simulink model "kwta2_block"  (R2024b)
settings: Solver=VariableStepAuto  StartTime=0.0  StopTime=2e-5  RelTol=1e-3
libraries: fl_lib x104, ee_lib x58, nesl_utility x13
(part 2 of 2)

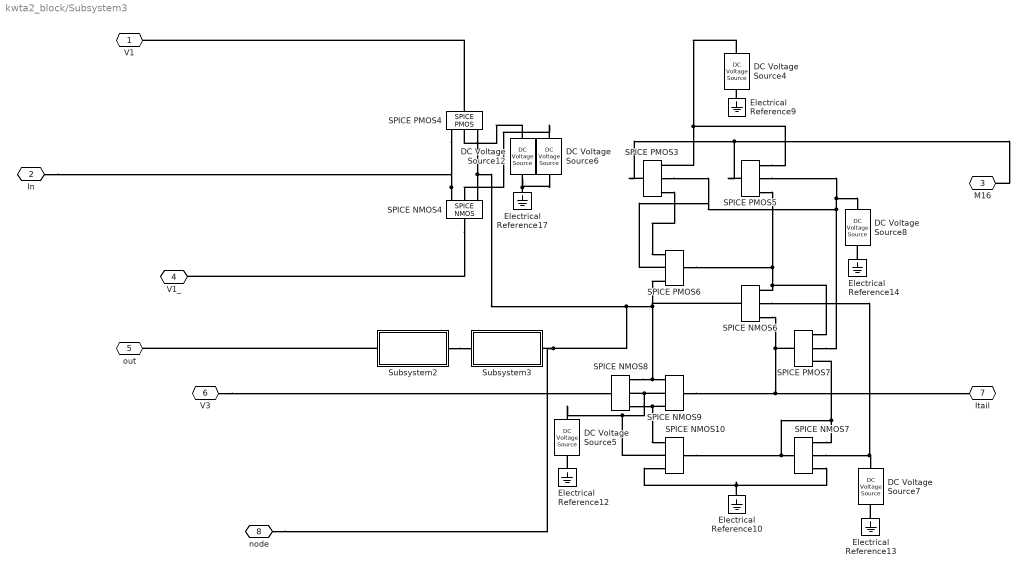
== system kwta2_block/Subsystem3 ==
  DC Voltage Source12 : fl_lib/Electrical/Electrical Sources/DC Voltage Source  v0=5 V
  DC Voltage Source4 : fl_lib/Electrical/Electrical Sources/DC Voltage Source  v0=5 V
  DC Voltage Source5 : fl_lib/Electrical/Electrical Sources/DC Voltage Source  v0=-5 V
  DC Voltage Source6 : fl_lib/Electrical/Electrical Sources/DC Voltage Source  v0=-5 V
  DC Voltage Source7 : fl_lib/Electrical/Electrical Sources/DC Voltage Source  v0=-5 V
  DC Voltage Source8 : fl_lib/Electrical/Electrical Sources/DC Voltage Source  v0=5 V
  Electrical Reference{9..10,12..14,17} (6 alike) : fl_lib/Electrical/Electrical Elements/Electrical Reference
  SPICE NMOS10 : ee_lib/Additional Components/SPICE Semiconductors/SPICE NMOS  LEVEL=3  AREA=1  SCALE=1  LENGTH=5 um  WIDTH=11 um  AD=0 m^2  AS=0 m^2  PD=0 m  PS=0 m  NRD=1  NRS=1  RD=0.01 Ohm  RS=1e-4 Ohm  RSH=NaN Ohm  VTO=0 V  KP=2e-5 A/V^2  GAMMA=0 V^0.50000  PHI=0.6 V  LAMBDA=0 1/V  IS=1e-14 A  N=1  JS=0 A/m^2  DELTA=0  VMAX=0 m/s  NFS=0 1/cm^2  ETA=0  THETA=0 1/V  KAPPA=0.2  Ci_param=ee.enum.intrinsicCapacitance.none  Cov_param=1  CGSO=0 F/m  CGDO=0 F/m  CGBO=0 F/m  C_param=1  CBD=0 F  CBS=0 F  PB=0.8 V  CJ=0 F/m^2  MJ=0.5  CJSW=0 F/m  MJSW=0.5  FC=0.5  IC_given=1  ICVDS=0 V  ICVGS=0 V  ICVBS=0 V  TOX=1e-7 m  LD=0 m  U0=600 cm^2/s/V  NSUB=NaN 1/cm^3  TPG=1  NSS=0 1/cm^2  XJ=0 m  T_param=1  TFIXED=300.15 K  TMEAS=300.15 K  TOFFSET=0 K  UEXP=0  UCRIT=1e+4 V/cm  NEFF=1  MTYPE=1
      settings: InternalSimscapePortConfiguration="{\"Bottom\":[],\"Left\":[{\"id\":\"gx\",\"label\":\"\",\"type\":\"foundation.electrical.electrical\"}],\"Right\":[{\"id\":\"dx\",\"label\":\"\",\"type\":\"foundation.electrical.electrical\"},{\"id\":\"bx\",\"label\":\"\",\"type\":\"foundation.electrical.electrical\"},{\"id\":\"sx\",\"label\":\"\",\"type\":\"foundation.electrical.electrical\"}],\"Top\":[]}"
  SPICE NMOS4 : ee_lib/Additional Components/SPICE Semiconductors/SPICE NMOS  LEVEL=3  AREA=1  SCALE=1  LENGTH=5 um  WIDTH=4 um  AD=0 m^2  AS=0 m^2  PD=0 m  PS=0 m  NRD=1  NRS=1  RD=0.01 Ohm  RS=1e-4 Ohm  RSH=NaN Ohm  VTO=0 V  KP=2e-5 A/V^2  GAMMA=0 V^0.50000  PHI=0.6 V  LAMBDA=0 1/V  IS=1e-14 A  N=1  JS=0 A/m^2  DELTA=0  VMAX=0 m/s  NFS=0 1/cm^2  ETA=0  THETA=0 1/V  KAPPA=0.2  Ci_param=ee.enum.intrinsicCapacitance.none  Cov_param=1  CGSO=0 F/m  CGDO=0 F/m  CGBO=0 F/m  C_param=1  CBD=0 F  CBS=0 F  PB=0.8 V  CJ=0 F/m^2  MJ=0.5  CJSW=0 F/m  MJSW=0.5  FC=0.5  IC_given=1  ICVDS=0 V  ICVGS=0 V  ICVBS=0 V  TOX=1e-7 m  LD=0 m  U0=600 cm^2/s/V  NSUB=NaN 1/cm^3  TPG=1  NSS=0 1/cm^2  XJ=0 m  T_param=1  TFIXED=300.15 K  TMEAS=300.15 K  TOFFSET=0 K  UEXP=0  UCRIT=1e+4 V/cm  NEFF=1  MTYPE=1
      settings: InternalSimscapePortConfiguration="{\"Bottom\":[],\"Left\":[{\"id\":\"gx\",\"label\":\"\",\"type\":\"foundation.electrical.electrical\"}],\"Right\":[{\"id\":\"dx\",\"label\":\"\",\"type\":\"foundation.electrical.electrical\"},{\"id\":\"bx\",\"label\":\"\",\"type\":\"foundation.electrical.electrical\"},{\"id\":\"sx\",\"label\":\"\",\"type\":\"foundation.electrical.electrical\"}],\"Top\":[]}"
  SPICE NMOS6 : ee_lib/Additional Components/SPICE Semiconductors/SPICE NMOS  LEVEL=3  AREA=1  SCALE=1  LENGTH=5 um  WIDTH=9 um  AD=0 m^2  AS=0 m^2  PD=0 m  PS=0 m  NRD=1  NRS=1  RD=0.01 Ohm  RS=1e-4 Ohm  RSH=NaN Ohm  VTO=0 V  KP=2e-5 A/V^2  GAMMA=0 V^0.50000  PHI=0.6 V  LAMBDA=0 1/V  IS=1e-14 A  N=1  JS=0 A/m^2  DELTA=0  VMAX=0 m/s  NFS=0 1/cm^2  ETA=0  THETA=0 1/V  KAPPA=0.2  Ci_param=ee.enum.intrinsicCapacitance.none  Cov_param=1  CGSO=0 F/m  CGDO=0 F/m  CGBO=0 F/m  C_param=1  CBD=0 F  CBS=0 F  PB=0.8 V  CJ=0 F/m^2  MJ=0.5  CJSW=0 F/m  MJSW=0.5  FC=0.5  IC_given=1  ICVDS=0 V  ICVGS=0 V  ICVBS=0 V  TOX=1e-7 m  LD=0 m  U0=600 cm^2/s/V  NSUB=NaN 1/cm^3  TPG=1  NSS=0 1/cm^2  XJ=0 m  T_param=1  TFIXED=300.15 K  TMEAS=300.15 K  TOFFSET=0 K  UEXP=0  UCRIT=1e+4 V/cm  NEFF=1  MTYPE=1
      settings: InternalSimscapePortConfiguration="{\"Bottom\":[],\"Left\":[{\"id\":\"gx\",\"label\":\"\",\"type\":\"foundation.electrical.electrical\"}],\"Right\":[{\"id\":\"dx\",\"label\":\"\",\"type\":\"foundation.electrical.electrical\"},{\"id\":\"bx\",\"label\":\"\",\"type\":\"foundation.electrical.electrical\"},{\"id\":\"sx\",\"label\":\"\",\"type\":\"foundation.electrical.electrical\"}],\"Top\":[]}"
  SPICE NMOS7 : ee_lib/Additional Components/SPICE Semiconductors/SPICE NMOS  LEVEL=3  AREA=1  SCALE=1  LENGTH=5 um  WIDTH=11 um  AD=0 m^2  AS=0 m^2  PD=0 m  PS=0 m  NRD=1  NRS=1  RD=0.01 Ohm  RS=1e-4 Ohm  RSH=NaN Ohm  VTO=0 V  KP=2e-5 A/V^2  GAMMA=0 V^0.50000  PHI=0.6 V  LAMBDA=0 1/V  IS=1e-14 A  N=1  JS=0 A/m^2  DELTA=0  VMAX=0 m/s  NFS=0 1/cm^2  ETA=0  THETA=0 1/V  KAPPA=0.2  Ci_param=ee.enum.intrinsicCapacitance.none  Cov_param=1  CGSO=0 F/m  CGDO=0 F/m  CGBO=0 F/m  C_param=1  CBD=0 F  CBS=0 F  PB=0.8 V  CJ=0 F/m^2  MJ=0.5  CJSW=0 F/m  MJSW=0.5  FC=0.5  IC_given=1  ICVDS=0 V  ICVGS=0 V  ICVBS=0 V  TOX=1e-7 m  LD=0 m  U0=600 cm^2/s/V  NSUB=NaN 1/cm^3  TPG=1  NSS=0 1/cm^2  XJ=0 m  T_param=1  TFIXED=300.15 K  TMEAS=300.15 K  TOFFSET=0 K  UEXP=0  UCRIT=1e+4 V/cm  NEFF=1  MTYPE=1
      settings: InternalSimscapePortConfiguration="{\"Bottom\":[],\"Left\":[{\"id\":\"gx\",\"label\":\"\",\"type\":\"foundation.electrical.electrical\"}],\"Right\":[{\"id\":\"dx\",\"label\":\"\",\"type\":\"foundation.electrical.electrical\"},{\"id\":\"bx\",\"label\":\"\",\"type\":\"foundation.electrical.electrical\"},{\"id\":\"sx\",\"label\":\"\",\"type\":\"foundation.electrical.electrical\"}],\"Top\":[]}"
  SPICE NMOS8 : ee_lib/Additional Components/SPICE Semiconductors/SPICE NMOS  LEVEL=3  AREA=1  SCALE=1  LENGTH=5 um  WIDTH=13 um  AD=0 m^2  AS=0 m^2  PD=0 m  PS=0 m  NRD=1  NRS=1  RD=0.01 Ohm  RS=1e-4 Ohm  RSH=NaN Ohm  VTO=0 V  KP=2e-5 A/V^2  GAMMA=0 V^0.50000  PHI=0.6 V  LAMBDA=0 1/V  IS=1e-14 A  N=1  JS=0 A/m^2  DELTA=0  VMAX=0 m/s  NFS=0 1/cm^2  ETA=0  THETA=0 1/V  KAPPA=0.2  Ci_param=ee.enum.intrinsicCapacitance.none  Cov_param=1  CGSO=0 F/m  CGDO=20 uF/m  CGBO=0 F/m  C_param=1  CBD=0 F  CBS=0 F  PB=0.8 V  CJ=0 F/m^2  MJ=0.5  CJSW=0 F/m  MJSW=0.5  FC=0.5  IC_given=1  ICVDS=0 V  ICVGS=0 V  ICVBS=0 V  TOX=1e-7 m  LD=0 m  U0=600 cm^2/s/V  NSUB=NaN 1/cm^3  TPG=1  NSS=0 1/cm^2  XJ=0 m  T_param=1  TFIXED=300.15 K  TMEAS=300.15 K  TOFFSET=0 K  UEXP=0  UCRIT=1e+4 V/cm  NEFF=1  MTYPE=1
      settings: InternalSimscapePortConfiguration="{\"Bottom\":[],\"Left\":[{\"id\":\"gx\",\"label\":\"\",\"type\":\"foundation.electrical.electrical\"}],\"Right\":[{\"id\":\"dx\",\"label\":\"\",\"type\":\"foundation.electrical.electrical\"},{\"id\":\"bx\",\"label\":\"\",\"type\":\"foundation.electrical.electrical\"},{\"id\":\"sx\",\"label\":\"\",\"type\":\"foundation.electrical.electrical\"}],\"Top\":[]}"
  SPICE NMOS9 : ee_lib/Additional Components/SPICE Semiconductors/SPICE NMOS  LEVEL=3  AREA=1  SCALE=1  LENGTH=5 um  WIDTH=13 um  AD=0 m^2  AS=0 m^2  PD=0 m  PS=0 m  NRD=1  NRS=1  RD=0.01 Ohm  RS=1e-4 Ohm  RSH=NaN Ohm  VTO=0 V  KP=2e-5 A/V^2  GAMMA=0 V^0.50000  PHI=0.6 V  LAMBDA=0 1/V  IS=1e-14 A  N=1  JS=0 A/m^2  DELTA=0  VMAX=0 m/s  NFS=0 1/cm^2  ETA=0  THETA=0 1/V  KAPPA=0.2  Ci_param=ee.enum.intrinsicCapacitance.none  Cov_param=2  CGSO=0 F/m  CGDO=1 uF/m  CGBO=0 F/m  C_param=2  CBD=0 F  CBS=0 F  PB=0.8 V  CJ=0 F/m^2  MJ=0.5  CJSW=0 F/m  MJSW=0.5  FC=0.5  IC_given=1  ICVDS=0 V  ICVGS=0 V  ICVBS=0 V  TOX=1e-7 m  LD=0 m  U0=600 cm^2/s/V  NSUB=NaN 1/cm^3  TPG=1  NSS=0 1/cm^2  XJ=0 m  T_param=1  TFIXED=300.15 K  TMEAS=300.15 K  TOFFSET=0 K  UEXP=0  UCRIT=1e+4 V/cm  NEFF=1  MTYPE=1
      settings: InternalSimscapePortConfiguration="{\"Bottom\":[],\"Left\":[{\"id\":\"gx\",\"label\":\"\",\"type\":\"foundation.electrical.electrical\"}],\"Right\":[{\"id\":\"dx\",\"label\":\"\",\"type\":\"foundation.electrical.electrical\"},{\"id\":\"bx\",\"label\":\"\",\"type\":\"foundation.electrical.electrical\"},{\"id\":\"sx\",\"label\":\"\",\"type\":\"foundation.electrical.electrical\"}],\"Top\":[]}"
  SPICE PMOS3 : ee_lib/Additional Components/SPICE Semiconductors/SPICE PMOS  LEVEL=3  AREA=1  SCALE=1  LENGTH=4 um  WIDTH=7 um  AD=0 m^2  AS=0 m^2  PD=0 m  PS=0 m  NRD=1  NRS=1  RD=0.01 Ohm  RS=1e-4 Ohm  RSH=NaN Ohm  VTO=0 V  KP=2e-5 A/V^2  GAMMA=0 V^0.50000  PHI=0.6 V  LAMBDA=0 1/V  IS=1e-14 A  N=1  JS=0 A/m^2  DELTA=0  VMAX=0 m/s  NFS=0 1/cm^2  ETA=0  THETA=0 1/V  KAPPA=0.2  Ci_param=ee.enum.intrinsicCapacitance.none  Cov_param=1  CGSO=0 F/m  CGDO=0 F/m  CGBO=0 F/m  C_param=1  CBD=0 F  CBS=0 F  PB=0.8 V  CJ=0 F/m^2  MJ=0.5  CJSW=0 F/m  MJSW=0.5  FC=0.5  IC_given=1  ICVDS=0 V  ICVGS=0 V  ICVBS=0 V  TOX=1e-7 m  LD=0 m  U0=600 cm^2/s/V  NSUB=NaN 1/cm^3  TPG=1  NSS=0 1/cm^2  XJ=0 m  T_param=1  TFIXED=300.15 K  TMEAS=300.15 K  TOFFSET=0 K  UEXP=0  UCRIT=1e+4 V/cm  NEFF=1  MTYPE=-1
      settings: InternalSimscapePortConfiguration="{\"Bottom\":[],\"Left\":[{\"id\":\"gx\",\"label\":\"\",\"type\":\"foundation.electrical.electrical\"}],\"Right\":[{\"id\":\"dx\",\"label\":\"\",\"type\":\"foundation.electrical.electrical\"},{\"id\":\"bx\",\"label\":\"\",\"type\":\"foundation.electrical.electrical\"},{\"id\":\"sx\",\"label\":\"\",\"type\":\"foundation.electrical.electrical\"}],\"Top\":[]}"
  SPICE PMOS4 : ee_lib/Additional Components/SPICE Semiconductors/SPICE PMOS  LEVEL=3  AREA=1  SCALE=1  LENGTH=5 um  WIDTH=4 um  AD=0 m^2  AS=0 m^2  PD=0 m  PS=0 m  NRD=1  NRS=1  RD=0.01 Ohm  RS=1e-4 Ohm  RSH=NaN Ohm  VTO=0 V  KP=2e-5 A/V^2  GAMMA=0 V^0.50000  PHI=0.6 V  LAMBDA=0 1/V  IS=1e-14 A  N=1  JS=0 A/m^2  DELTA=0  VMAX=0 m/s  NFS=0 1/cm^2  ETA=0  THETA=0 1/V  KAPPA=0.2  Ci_param=ee.enum.intrinsicCapacitance.none  Cov_param=1  CGSO=0 F/m  CGDO=0 F/m  CGBO=0 F/m  C_param=1  CBD=0 F  CBS=0 F  PB=0.8 V  CJ=0 F/m^2  MJ=0.5  CJSW=0 F/m  MJSW=0.5  FC=0.5  IC_given=1  ICVDS=0 V  ICVGS=0 V  ICVBS=0 V  TOX=1e-7 m  LD=0 m  U0=600 cm^2/s/V  NSUB=NaN 1/cm^3  TPG=1  NSS=0 1/cm^2  XJ=0 m  T_param=1  TFIXED=300.15 K  TMEAS=300.15 K  TOFFSET=0 K  UEXP=0  UCRIT=1e+4 V/cm  NEFF=1  MTYPE=-1
      settings: InternalSimscapePortConfiguration="{\"Bottom\":[],\"Left\":[{\"id\":\"gx\",\"label\":\"\",\"type\":\"foundation.electrical.electrical\"}],\"Right\":[{\"id\":\"dx\",\"label\":\"\",\"type\":\"foundation.electrical.electrical\"},{\"id\":\"bx\",\"label\":\"\",\"type\":\"foundation.electrical.electrical\"},{\"id\":\"sx\",\"label\":\"\",\"type\":\"foundation.electrical.electrical\"}],\"Top\":[]}"
  SPICE PMOS5 : ee_lib/Additional Components/SPICE Semiconductors/SPICE PMOS  LEVEL=3  AREA=1  SCALE=1  LENGTH=4 um  WIDTH=21 um  AD=0 m^2  AS=0 m^2  PD=0 m  PS=0 m  NRD=1  NRS=1  RD=0.01 Ohm  RS=1e-4 Ohm  RSH=NaN Ohm  VTO=0 V  KP=2e-5 A/V^2  GAMMA=0 V^0.50000  PHI=0.6 V  LAMBDA=0 1/V  IS=1e-14 A  N=1  JS=0 A/m^2  DELTA=0  VMAX=0 m/s  NFS=0 1/cm^2  ETA=0  THETA=0 1/V  KAPPA=0.2  Ci_param=ee.enum.intrinsicCapacitance.none  Cov_param=1  CGSO=0 F/m  CGDO=0 F/m  CGBO=0 F/m  C_param=1  CBD=0 F  CBS=0 F  PB=0.8 V  CJ=0 F/m^2  MJ=0.5  CJSW=0 F/m  MJSW=0.5  FC=0.5  IC_given=1  ICVDS=0 V  ICVGS=0 V  ICVBS=0 V  TOX=1e-7 m  LD=0 m  U0=600 cm^2/s/V  NSUB=NaN 1/cm^3  TPG=1  NSS=0 1/cm^2  XJ=0 m  T_param=1  TFIXED=300.15 K  TMEAS=300.15 K  TOFFSET=0 K  UEXP=0  UCRIT=1e+4 V/cm  NEFF=1  MTYPE=-1
      settings: InternalSimscapePortConfiguration="{\"Bottom\":[],\"Left\":[{\"id\":\"gx\",\"label\":\"\",\"type\":\"foundation.electrical.electrical\"}],\"Right\":[{\"id\":\"dx\",\"label\":\"\",\"type\":\"foundation.electrical.electrical\"},{\"id\":\"bx\",\"label\":\"\",\"type\":\"foundation.electrical.electrical\"},{\"id\":\"sx\",\"label\":\"\",\"type\":\"foundation.electrical.electrical\"}],\"Top\":[]}"
  SPICE PMOS6 : ee_lib/Additional Components/SPICE Semiconductors/SPICE PMOS  LEVEL=3  AREA=1  SCALE=1  LENGTH=4 um  WIDTH=7 um  AD=0 m^2  AS=0 m^2  PD=0 m  PS=0 m  NRD=1  NRS=1  RD=0.01 Ohm  RS=1e-4 Ohm  RSH=NaN Ohm  VTO=0 V  KP=2e-5 A/V^2  GAMMA=0 V^0.50000  PHI=0.6 V  LAMBDA=0 1/V  IS=1e-14 A  N=1  JS=0 A/m^2  DELTA=0  VMAX=0 m/s  NFS=0 1/cm^2  ETA=0  THETA=0 1/V  KAPPA=0.2  Ci_param=ee.enum.intrinsicCapacitance.none  Cov_param=1  CGSO=0 F/m  CGDO=0 F/m  CGBO=0 F/m  C_param=1  CBD=0 F  CBS=0 F  PB=0.8 V  CJ=0 F/m^2  MJ=0.5  CJSW=0 F/m  MJSW=0.5  FC=0.5  IC_given=1  ICVDS=0 V  ICVGS=0 V  ICVBS=0 V  TOX=1e-7 m  LD=0 m  U0=600 cm^2/s/V  NSUB=NaN 1/cm^3  TPG=1  NSS=0 1/cm^2  XJ=0 m  T_param=1  TFIXED=300.15 K  TMEAS=300.15 K  TOFFSET=0 K  UEXP=0  UCRIT=1e+4 V/cm  NEFF=1  MTYPE=-1
      settings: InternalSimscapePortConfiguration="{\"Bottom\":[],\"Left\":[{\"id\":\"gx\",\"label\":\"\",\"type\":\"foundation.electrical.electrical\"}],\"Right\":[{\"id\":\"dx\",\"label\":\"\",\"type\":\"foundation.electrical.electrical\"},{\"id\":\"bx\",\"label\":\"\",\"type\":\"foundation.electrical.electrical\"},{\"id\":\"sx\",\"label\":\"\",\"type\":\"foundation.electrical.electrical\"}],\"Top\":[]}"
  SPICE PMOS7 : ee_lib/Additional Components/SPICE Semiconductors/SPICE PMOS  LEVEL=3  AREA=1  SCALE=1  LENGTH=4 um  WIDTH=17 um  AD=0 m^2  AS=0 m^2  PD=0 m  PS=0 m  NRD=1  NRS=1  RD=0.01 Ohm  RS=1e-4 Ohm  RSH=NaN Ohm  VTO=0 V  KP=2e-5 A/V^2  GAMMA=0 V^0.50000  PHI=0.6 V  LAMBDA=0 1/V  IS=1e-14 A  N=1  JS=0 A/m^2  DELTA=0  VMAX=0 m/s  NFS=0 1/cm^2  ETA=0  THETA=0 1/V  KAPPA=0.2  Ci_param=ee.enum.intrinsicCapacitance.none  Cov_param=1  CGSO=0 F/m  CGDO=0 F/m  CGBO=0 F/m  C_param=1  CBD=0 F  CBS=0 F  PB=0.8 V  CJ=0 F/m^2  MJ=0.5  CJSW=0 F/m  MJSW=0.5  FC=0.5  IC_given=1  ICVDS=0 V  ICVGS=0 V  ICVBS=0 V  TOX=1e-7 m  LD=0 m  U0=600 cm^2/s/V  NSUB=NaN 1/cm^3  TPG=1  NSS=0 1/cm^2  XJ=0 m  T_param=1  TFIXED=300.15 K  TMEAS=300.15 K  TOFFSET=0 K  UEXP=0  UCRIT=1e+4 V/cm  NEFF=1  MTYPE=-1
      settings: InternalSimscapePortConfiguration="{\"Bottom\":[],\"Left\":[{\"id\":\"gx\",\"label\":\"\",\"type\":\"foundation.electrical.electrical\"}],\"Right\":[{\"id\":\"dx\",\"label\":\"\",\"type\":\"foundation.electrical.electrical\"},{\"id\":\"bx\",\"label\":\"\",\"type\":\"foundation.electrical.electrical\"},{\"id\":\"sx\",\"label\":\"\",\"type\":\"foundation.electrical.electrical\"}],\"Top\":[]}"
  Subsystem2 : Subsystem
  Subsystem3 : Subsystem
  V1 : PMIOPort  Side=Left
  In : PMIOPort  Port=2  Side=Left
  M16 : PMIOPort  Port=3  Side=Right
  V1_ : PMIOPort  Port=4  Side=Left
  out : PMIOPort  Port=5  Side=Left
  V3 : PMIOPort  Port=6  Side=Left
  Itail : PMIOPort  Port=7  Side=Right
  "node " : PMIOPort  Port=8  Side=Left
  connections:
  SPICE NMOS6/RConn3 -- Itail/RConn1 -- SPICE NMOS9/LConn1 -- SPICE PMOS7/LConn1
  SPICE PMOS5/RConn3 -- SPICE PMOS6/LConn1 -- SPICE PMOS7/RConn1 -- SPICE NMOS6/RConn1
  Electrical Reference10/LConn1 -- SPICE NMOS10/RConn3 -- SPICE NMOS7/RConn3
  Subsystem2/LConn1 -- out/RConn1
  DC Voltage Source4/LConn1 -- SPICE PMOS3/RConn1 -- SPICE PMOS5/RConn1
  DC Voltage Source6/LConn1 -- SPICE NMOS4/RConn2
  V3/RConn1 -- SPICE NMOS8/LConn1
  DC Voltage Source12/LConn1 -- SPICE PMOS4/RConn2
  DC Voltage Source5/LConn1 -- SPICE NMOS10/RConn2 -- SPICE NMOS9/RConn2 -- SPICE NMOS8/RConn2
  DC Voltage Source12/RConn1 -- DC Voltage Source6/RConn1 -- Electrical Reference17/LConn1
  SPICE NMOS4/RConn1 -- SPICE PMOS4/RConn3 -- In/RConn1
  SPICE PMOS5/LConn1 -- M16/RConn1 -- SPICE PMOS3/LConn1
  SPICE PMOS4/LConn1 -- V1/RConn1
  Electrical Reference9/LConn1 -- DC Voltage Source4/RConn1
  Electrical Reference14/LConn1 -- DC Voltage Source8/RConn1
  SPICE PMOS7/RConn2 -- SPICE PMOS3/RConn2 -- SPICE PMOS6/RConn2 -- SPICE PMOS5/RConn2 -- DC Voltage Source8/LConn1
  SPICE PMOS3/RConn3 -- SPICE PMOS6/RConn1
  SPICE NMOS10/LConn1 -- SPICE PMOS7/RConn3 -- SPICE NMOS7/RConn1 -- SPICE NMOS7/LConn1
  SPICE PMOS4/RConn1 -- SPICE NMOS4/RConn3 -- "node "/RConn1 -- Subsystem3/RConn1 -- SPICE PMOS6/RConn3 -- SPICE NMOS6/LConn1 -- SPICE NMOS8/RConn1 -- SPICE NMOS9/RConn1
  SPICE NMOS7/RConn2 -- SPICE NMOS6/RConn2 -- DC Voltage Source7/LConn1
  SPICE NMOS9/RConn3 -- SPICE NMOS8/RConn3 -- SPICE NMOS10/RConn1
  Subsystem2/RConn1 -- Subsystem3/LConn1
  SPICE NMOS4/LConn1 -- V1_/RConn1
  Electrical Reference13/LConn1 -- DC Voltage Source7/RConn1
  Electrical Reference12/LConn1 -- DC Voltage Source5/RConn1

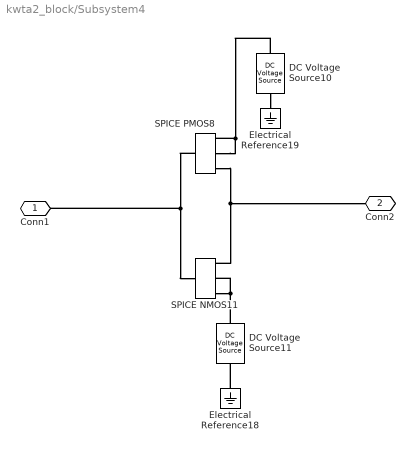
== system kwta2_block/Subsystem4 ==
  DC Voltage Source10 : fl_lib/Electrical/Electrical Sources/DC Voltage Source  v0=5 V
  DC Voltage Source11 : fl_lib/Electrical/Electrical Sources/DC Voltage Source  v0=0 V
  Electrical Reference18 : fl_lib/Electrical/Electrical Elements/Electrical Reference
  Electrical Reference19 : fl_lib/Electrical/Electrical Elements/Electrical Reference
  SPICE NMOS11 : ee_lib/Additional Components/SPICE Semiconductors/SPICE NMOS  LEVEL=1  AREA=1  SCALE=1  LENGTH=1e-4 mm  WIDTH=1e-4 mm  AD=0 m^2  AS=0 m^2  PD=0 m  PS=0 m  NRD=1  NRS=1  RD=0.01 Ohm  RS=1e-4 Ohm  RSH=NaN Ohm  VTO=0 V  KP=2e-5 A/V^2  GAMMA=0 V^0.50000  PHI=0.6 V  LAMBDA=0 1/V  IS=1e-14 A  N=1  JS=0 A/m^2  DELTA=0  VMAX=0 m/s  NFS=0 1/cm^2  ETA=0  THETA=0 1/V  KAPPA=0.2  Ci_param=ee.enum.intrinsicCapacitance.none  Cov_param=1  CGSO=0 F/m  CGDO=0 F/m  CGBO=0 F/m  C_param=1  CBD=0 F  CBS=0 F  PB=0.8 V  CJ=0 F/m^2  MJ=0.5  CJSW=0 F/m  MJSW=0.5  FC=0.5  IC_given=1  ICVDS=0 V  ICVGS=0 V  ICVBS=0 V  TOX=1e-7 m  LD=0 m  U0=600 cm^2/s/V  NSUB=NaN 1/cm^3  TPG=1  NSS=0 1/cm^2  XJ=0 m  T_param=1  TFIXED=300.15 K  TMEAS=300.15 K  TOFFSET=0 K  UEXP=0  UCRIT=1e+4 V/cm  NEFF=1  MTYPE=1
      settings: InternalSimscapePortConfiguration="{\"Bottom\":[],\"Left\":[{\"id\":\"gx\",\"label\":\"\",\"type\":\"foundation.electrical.electrical\"}],\"Right\":[{\"id\":\"dx\",\"label\":\"\",\"type\":\"foundation.electrical.electrical\"},{\"id\":\"bx\",\"label\":\"\",\"type\":\"foundation.electrical.electrical\"},{\"id\":\"sx\",\"label\":\"\",\"type\":\"foundation.electrical.electrical\"}],\"Top\":[]}"
  SPICE PMOS8 : ee_lib/Additional Components/SPICE Semiconductors/SPICE PMOS  LEVEL=1  AREA=1  SCALE=1  LENGTH=1e-4 mm  WIDTH=1e-4 mm  AD=0 m^2  AS=0 m^2  PD=0 m  PS=0 m  NRD=1  NRS=1  RD=0.01 Ohm  RS=1e-4 Ohm  RSH=NaN Ohm  VTO=0 V  KP=2e-5 A/V^2  GAMMA=0 V^0.50000  PHI=0.6 V  LAMBDA=0 1/V  IS=1e-14 A  N=1  JS=0 A/m^2  DELTA=0  VMAX=0 m/s  NFS=0 1/cm^2  ETA=0  THETA=0 1/V  KAPPA=0.2  Ci_param=ee.enum.intrinsicCapacitance.none  Cov_param=1  CGSO=0 F/m  CGDO=0 F/m  CGBO=0 F/m  C_param=1  CBD=0 F  CBS=0 F  PB=0.8 V  CJ=0 F/m^2  MJ=0.5  CJSW=0 F/m  MJSW=0.5  FC=0.5  IC_given=1  ICVDS=0 V  ICVGS=0 V  ICVBS=0 V  TOX=1e-7 m  LD=0 m  U0=600 cm^2/s/V  NSUB=NaN 1/cm^3  TPG=1  NSS=0 1/cm^2  XJ=0 m  T_param=1  TFIXED=300.15 K  TMEAS=300.15 K  TOFFSET=0 K  UEXP=0  UCRIT=1e+4 V/cm  NEFF=1  MTYPE=-1
      settings: InternalSimscapePortConfiguration="{\"Bottom\":[],\"Left\":[{\"id\":\"gx\",\"label\":\"\",\"type\":\"foundation.electrical.electrical\"}],\"Right\":[{\"id\":\"dx\",\"label\":\"\",\"type\":\"foundation.electrical.electrical\"},{\"id\":\"bx\",\"label\":\"\",\"type\":\"foundation.electrical.electrical\"},{\"id\":\"sx\",\"label\":\"\",\"type\":\"foundation.electrical.electrical\"}],\"Top\":[]}"
  Conn1 : PMIOPort  Side=Right
  Conn2 : PMIOPort  Port=2  Side=Left
  connections:
  DC Voltage Source10/RConn1 -- Electrical Reference19/LConn1
  SPICE NMOS11/RConn1 -- Conn2/RConn1 -- SPICE PMOS8/RConn3
  Electrical Reference18/LConn1 -- DC Voltage Source11/RConn1
  DC Voltage Source11/LConn1 -- SPICE NMOS11/RConn2 -- SPICE NMOS11/RConn3
  DC Voltage Source10/LConn1 -- SPICE PMOS8/RConn1 -- SPICE PMOS8/RConn2
  Conn1/RConn1 -- SPICE NMOS11/LConn1 -- SPICE PMOS8/LConn1

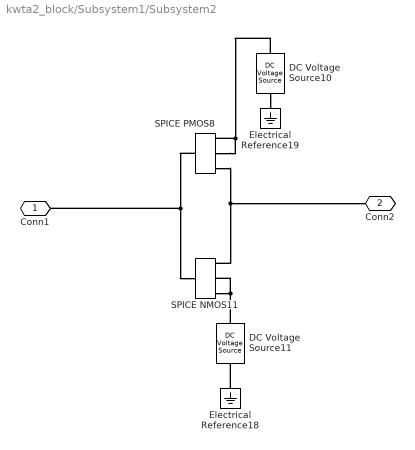
== system kwta2_block/Subsystem1/Subsystem2 ==
  DC Voltage Source10 : fl_lib/Electrical/Electrical Sources/DC Voltage Source  v0=5 V
  DC Voltage Source11 : fl_lib/Electrical/Electrical Sources/DC Voltage Source  v0=0 V
  Electrical Reference18 : fl_lib/Electrical/Electrical Elements/Electrical Reference
  Electrical Reference19 : fl_lib/Electrical/Electrical Elements/Electrical Reference
  SPICE NMOS11 : ee_lib/Additional Components/SPICE Semiconductors/SPICE NMOS  LEVEL=1  AREA=1  SCALE=1  LENGTH=1e-4 mm  WIDTH=1e-4 mm  AD=0 m^2  AS=0 m^2  PD=0 m  PS=0 m  NRD=1  NRS=1  RD=0.01 Ohm  RS=1e-4 Ohm  RSH=NaN Ohm  VTO=0 V  KP=2e-5 A/V^2  GAMMA=0 V^0.50000  PHI=0.6 V  LAMBDA=0 1/V  IS=1e-14 A  N=1  JS=0 A/m^2  DELTA=0  VMAX=0 m/s  NFS=0 1/cm^2  ETA=0  THETA=0 1/V  KAPPA=0.2  Ci_param=ee.enum.intrinsicCapacitance.none  Cov_param=1  CGSO=0 F/m  CGDO=0 F/m  CGBO=0 F/m  C_param=1  CBD=0 F  CBS=0 F  PB=0.8 V  CJ=0 F/m^2  MJ=0.5  CJSW=0 F/m  MJSW=0.5  FC=0.5  IC_given=1  ICVDS=0 V  ICVGS=0 V  ICVBS=0 V  TOX=1e-7 m  LD=0 m  U0=600 cm^2/s/V  NSUB=NaN 1/cm^3  TPG=1  NSS=0 1/cm^2  XJ=0 m  T_param=1  TFIXED=300.15 K  TMEAS=300.15 K  TOFFSET=0 K  UEXP=0  UCRIT=1e+4 V/cm  NEFF=1  MTYPE=1
      settings: InternalSimscapePortConfiguration="{\"Bottom\":[],\"Left\":[{\"id\":\"gx\",\"label\":\"\",\"type\":\"foundation.electrical.electrical\"}],\"Right\":[{\"id\":\"dx\",\"label\":\"\",\"type\":\"foundation.electrical.electrical\"},{\"id\":\"bx\",\"label\":\"\",\"type\":\"foundation.electrical.electrical\"},{\"id\":\"sx\",\"label\":\"\",\"type\":\"foundation.electrical.electrical\"}],\"Top\":[]}"
  SPICE PMOS8 : ee_lib/Additional Components/SPICE Semiconductors/SPICE PMOS  LEVEL=1  AREA=1  SCALE=1  LENGTH=1e-4 mm  WIDTH=1e-4 mm  AD=0 m^2  AS=0 m^2  PD=0 m  PS=0 m  NRD=1  NRS=1  RD=0.01 Ohm  RS=1e-4 Ohm  RSH=NaN Ohm  VTO=0 V  KP=2e-5 A/V^2  GAMMA=0 V^0.50000  PHI=0.6 V  LAMBDA=0 1/V  IS=1e-14 A  N=1  JS=0 A/m^2  DELTA=0  VMAX=0 m/s  NFS=0 1/cm^2  ETA=0  THETA=0 1/V  KAPPA=0.2  Ci_param=ee.enum.intrinsicCapacitance.none  Cov_param=1  CGSO=0 F/m  CGDO=0 F/m  CGBO=0 F/m  C_param=1  CBD=0 F  CBS=0 F  PB=0.8 V  CJ=0 F/m^2  MJ=0.5  CJSW=0 F/m  MJSW=0.5  FC=0.5  IC_given=1  ICVDS=0 V  ICVGS=0 V  ICVBS=0 V  TOX=1e-7 m  LD=0 m  U0=600 cm^2/s/V  NSUB=NaN 1/cm^3  TPG=1  NSS=0 1/cm^2  XJ=0 m  T_param=1  TFIXED=300.15 K  TMEAS=300.15 K  TOFFSET=0 K  UEXP=0  UCRIT=1e+4 V/cm  NEFF=1  MTYPE=-1
      settings: InternalSimscapePortConfiguration="{\"Bottom\":[],\"Left\":[{\"id\":\"gx\",\"label\":\"\",\"type\":\"foundation.electrical.electrical\"}],\"Right\":[{\"id\":\"dx\",\"label\":\"\",\"type\":\"foundation.electrical.electrical\"},{\"id\":\"bx\",\"label\":\"\",\"type\":\"foundation.electrical.electrical\"},{\"id\":\"sx\",\"label\":\"\",\"type\":\"foundation.electrical.electrical\"}],\"Top\":[]}"
  Conn1 : PMIOPort  Side=Right
  Conn2 : PMIOPort  Port=2  Side=Left
  connections:
  DC Voltage Source10/RConn1 -- Electrical Reference19/LConn1
  SPICE NMOS11/RConn1 -- Conn2/RConn1 -- SPICE PMOS8/RConn3
  Electrical Reference18/LConn1 -- DC Voltage Source11/RConn1
  DC Voltage Source11/LConn1 -- SPICE NMOS11/RConn2 -- SPICE NMOS11/RConn3
  DC Voltage Source10/LConn1 -- SPICE PMOS8/RConn1 -- SPICE PMOS8/RConn2
  Conn1/RConn1 -- SPICE NMOS11/LConn1 -- SPICE PMOS8/LConn1

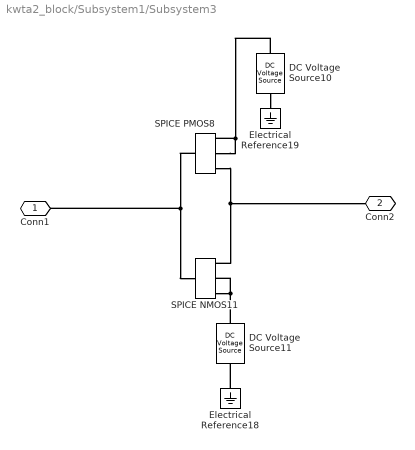
== system kwta2_block/Subsystem1/Subsystem3 ==
  DC Voltage Source10 : fl_lib/Electrical/Electrical Sources/DC Voltage Source  v0=5 V
  DC Voltage Source11 : fl_lib/Electrical/Electrical Sources/DC Voltage Source  v0=0 V
  Electrical Reference18 : fl_lib/Electrical/Electrical Elements/Electrical Reference
  Electrical Reference19 : fl_lib/Electrical/Electrical Elements/Electrical Reference
  SPICE NMOS11 : ee_lib/Additional Components/SPICE Semiconductors/SPICE NMOS  LEVEL=1  AREA=1  SCALE=1  LENGTH=1e-4 mm  WIDTH=1e-4 mm  AD=0 m^2  AS=0 m^2  PD=0 m  PS=0 m  NRD=1  NRS=1  RD=0.01 Ohm  RS=1e-4 Ohm  RSH=NaN Ohm  VTO=0 V  KP=2e-5 A/V^2  GAMMA=0 V^0.50000  PHI=0.6 V  LAMBDA=0 1/V  IS=1e-14 A  N=1  JS=0 A/m^2  DELTA=0  VMAX=0 m/s  NFS=0 1/cm^2  ETA=0  THETA=0 1/V  KAPPA=0.2  Ci_param=ee.enum.intrinsicCapacitance.none  Cov_param=1  CGSO=0 F/m  CGDO=0 F/m  CGBO=0 F/m  C_param=1  CBD=0 F  CBS=0 F  PB=0.8 V  CJ=0 F/m^2  MJ=0.5  CJSW=0 F/m  MJSW=0.5  FC=0.5  IC_given=1  ICVDS=0 V  ICVGS=0 V  ICVBS=0 V  TOX=1e-7 m  LD=0 m  U0=600 cm^2/s/V  NSUB=NaN 1/cm^3  TPG=1  NSS=0 1/cm^2  XJ=0 m  T_param=1  TFIXED=300.15 K  TMEAS=300.15 K  TOFFSET=0 K  UEXP=0  UCRIT=1e+4 V/cm  NEFF=1  MTYPE=1
      settings: InternalSimscapePortConfiguration="{\"Bottom\":[],\"Left\":[{\"id\":\"gx\",\"label\":\"\",\"type\":\"foundation.electrical.electrical\"}],\"Right\":[{\"id\":\"dx\",\"label\":\"\",\"type\":\"foundation.electrical.electrical\"},{\"id\":\"bx\",\"label\":\"\",\"type\":\"foundation.electrical.electrical\"},{\"id\":\"sx\",\"label\":\"\",\"type\":\"foundation.electrical.electrical\"}],\"Top\":[]}"
  SPICE PMOS8 : ee_lib/Additional Components/SPICE Semiconductors/SPICE PMOS  LEVEL=1  AREA=1  SCALE=1  LENGTH=1e-4 mm  WIDTH=1e-4 mm  AD=0 m^2  AS=0 m^2  PD=0 m  PS=0 m  NRD=1  NRS=1  RD=0.01 Ohm  RS=1e-4 Ohm  RSH=NaN Ohm  VTO=0 V  KP=2e-5 A/V^2  GAMMA=0 V^0.50000  PHI=0.6 V  LAMBDA=0 1/V  IS=1e-14 A  N=1  JS=0 A/m^2  DELTA=0  VMAX=0 m/s  NFS=0 1/cm^2  ETA=0  THETA=0 1/V  KAPPA=0.2  Ci_param=ee.enum.intrinsicCapacitance.none  Cov_param=1  CGSO=0 F/m  CGDO=0 F/m  CGBO=0 F/m  C_param=1  CBD=0 F  CBS=0 F  PB=0.8 V  CJ=0 F/m^2  MJ=0.5  CJSW=0 F/m  MJSW=0.5  FC=0.5  IC_given=1  ICVDS=0 V  ICVGS=0 V  ICVBS=0 V  TOX=1e-7 m  LD=0 m  U0=600 cm^2/s/V  NSUB=NaN 1/cm^3  TPG=1  NSS=0 1/cm^2  XJ=0 m  T_param=1  TFIXED=300.15 K  TMEAS=300.15 K  TOFFSET=0 K  UEXP=0  UCRIT=1e+4 V/cm  NEFF=1  MTYPE=-1
      settings: InternalSimscapePortConfiguration="{\"Bottom\":[],\"Left\":[{\"id\":\"gx\",\"label\":\"\",\"type\":\"foundation.electrical.electrical\"}],\"Right\":[{\"id\":\"dx\",\"label\":\"\",\"type\":\"foundation.electrical.electrical\"},{\"id\":\"bx\",\"label\":\"\",\"type\":\"foundation.electrical.electrical\"},{\"id\":\"sx\",\"label\":\"\",\"type\":\"foundation.electrical.electrical\"}],\"Top\":[]}"
  Conn1 : PMIOPort  Side=Right
  Conn2 : PMIOPort  Port=2  Side=Left
  connections:
  SPICE PMOS8/LConn1 -- SPICE NMOS11/LConn1 -- Conn1/RConn1
  SPICE PMOS8/RConn2 -- SPICE PMOS8/RConn1 -- DC Voltage Source10/LConn1
  SPICE NMOS11/RConn3 -- SPICE NMOS11/RConn2 -- DC Voltage Source11/LConn1
  Electrical Reference18/LConn1 -- DC Voltage Source11/RConn1
  SPICE PMOS8/RConn3 -- Conn2/RConn1 -- SPICE NMOS11/RConn1
  DC Voltage Source10/RConn1 -- Electrical Reference19/LConn1

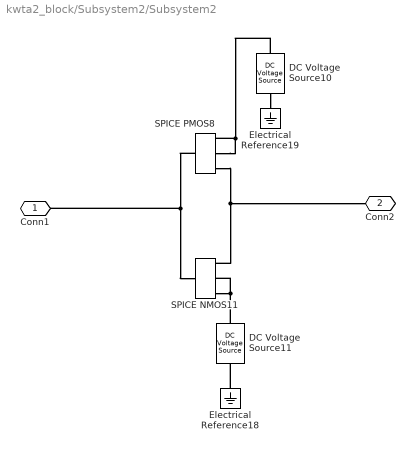
== system kwta2_block/Subsystem2/Subsystem2 ==
  DC Voltage Source10 : fl_lib/Electrical/Electrical Sources/DC Voltage Source  v0=5 V
  DC Voltage Source11 : fl_lib/Electrical/Electrical Sources/DC Voltage Source  v0=0 V
  Electrical Reference18 : fl_lib/Electrical/Electrical Elements/Electrical Reference
  Electrical Reference19 : fl_lib/Electrical/Electrical Elements/Electrical Reference
  SPICE NMOS11 : ee_lib/Additional Components/SPICE Semiconductors/SPICE NMOS  LEVEL=1  AREA=1  SCALE=1  LENGTH=1e-4 mm  WIDTH=1e-4 mm  AD=0 m^2  AS=0 m^2  PD=0 m  PS=0 m  NRD=1  NRS=1  RD=0.01 Ohm  RS=1e-4 Ohm  RSH=NaN Ohm  VTO=0 V  KP=2e-5 A/V^2  GAMMA=0 V^0.50000  PHI=0.6 V  LAMBDA=0 1/V  IS=1e-14 A  N=1  JS=0 A/m^2  DELTA=0  VMAX=0 m/s  NFS=0 1/cm^2  ETA=0  THETA=0 1/V  KAPPA=0.2  Ci_param=ee.enum.intrinsicCapacitance.none  Cov_param=1  CGSO=0 F/m  CGDO=0 F/m  CGBO=0 F/m  C_param=1  CBD=0 F  CBS=0 F  PB=0.8 V  CJ=0 F/m^2  MJ=0.5  CJSW=0 F/m  MJSW=0.5  FC=0.5  IC_given=1  ICVDS=0 V  ICVGS=0 V  ICVBS=0 V  TOX=1e-7 m  LD=0 m  U0=600 cm^2/s/V  NSUB=NaN 1/cm^3  TPG=1  NSS=0 1/cm^2  XJ=0 m  T_param=1  TFIXED=300.15 K  TMEAS=300.15 K  TOFFSET=0 K  UEXP=0  UCRIT=1e+4 V/cm  NEFF=1  MTYPE=1
      settings: InternalSimscapePortConfiguration="{\"Bottom\":[],\"Left\":[{\"id\":\"gx\",\"label\":\"\",\"type\":\"foundation.electrical.electrical\"}],\"Right\":[{\"id\":\"dx\",\"label\":\"\",\"type\":\"foundation.electrical.electrical\"},{\"id\":\"bx\",\"label\":\"\",\"type\":\"foundation.electrical.electrical\"},{\"id\":\"sx\",\"label\":\"\",\"type\":\"foundation.electrical.electrical\"}],\"Top\":[]}"
  SPICE PMOS8 : ee_lib/Additional Components/SPICE Semiconductors/SPICE PMOS  LEVEL=1  AREA=1  SCALE=1  LENGTH=1e-4 mm  WIDTH=1e-4 mm  AD=0 m^2  AS=0 m^2  PD=0 m  PS=0 m  NRD=1  NRS=1  RD=0.01 Ohm  RS=1e-4 Ohm  RSH=NaN Ohm  VTO=0 V  KP=2e-5 A/V^2  GAMMA=0 V^0.50000  PHI=0.6 V  LAMBDA=0 1/V  IS=1e-14 A  N=1  JS=0 A/m^2  DELTA=0  VMAX=0 m/s  NFS=0 1/cm^2  ETA=0  THETA=0 1/V  KAPPA=0.2  Ci_param=ee.enum.intrinsicCapacitance.none  Cov_param=1  CGSO=0 F/m  CGDO=0 F/m  CGBO=0 F/m  C_param=1  CBD=0 F  CBS=0 F  PB=0.8 V  CJ=0 F/m^2  MJ=0.5  CJSW=0 F/m  MJSW=0.5  FC=0.5  IC_given=1  ICVDS=0 V  ICVGS=0 V  ICVBS=0 V  TOX=1e-7 m  LD=0 m  U0=600 cm^2/s/V  NSUB=NaN 1/cm^3  TPG=1  NSS=0 1/cm^2  XJ=0 m  T_param=1  TFIXED=300.15 K  TMEAS=300.15 K  TOFFSET=0 K  UEXP=0  UCRIT=1e+4 V/cm  NEFF=1  MTYPE=-1
      settings: InternalSimscapePortConfiguration="{\"Bottom\":[],\"Left\":[{\"id\":\"gx\",\"label\":\"\",\"type\":\"foundation.electrical.electrical\"}],\"Right\":[{\"id\":\"dx\",\"label\":\"\",\"type\":\"foundation.electrical.electrical\"},{\"id\":\"bx\",\"label\":\"\",\"type\":\"foundation.electrical.electrical\"},{\"id\":\"sx\",\"label\":\"\",\"type\":\"foundation.electrical.electrical\"}],\"Top\":[]}"
  Conn1 : PMIOPort  Side=Right
  Conn2 : PMIOPort  Port=2  Side=Left
  connections:
  SPICE PMOS8/LConn1 -- SPICE NMOS11/LConn1 -- Conn1/RConn1
  SPICE PMOS8/RConn2 -- SPICE PMOS8/RConn1 -- DC Voltage Source10/LConn1
  SPICE NMOS11/RConn3 -- SPICE NMOS11/RConn2 -- DC Voltage Source11/LConn1
  Electrical Reference18/LConn1 -- DC Voltage Source11/RConn1
  SPICE PMOS8/RConn3 -- Conn2/RConn1 -- SPICE NMOS11/RConn1
  DC Voltage Source10/RConn1 -- Electrical Reference19/LConn1

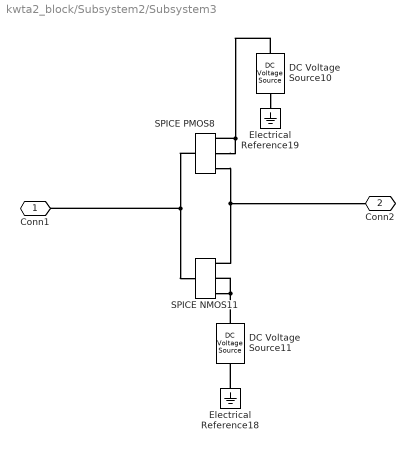
== system kwta2_block/Subsystem2/Subsystem3 ==
  DC Voltage Source10 : fl_lib/Electrical/Electrical Sources/DC Voltage Source  v0=5 V
  DC Voltage Source11 : fl_lib/Electrical/Electrical Sources/DC Voltage Source  v0=0 V
  Electrical Reference18 : fl_lib/Electrical/Electrical Elements/Electrical Reference
  Electrical Reference19 : fl_lib/Electrical/Electrical Elements/Electrical Reference
  SPICE NMOS11 : ee_lib/Additional Components/SPICE Semiconductors/SPICE NMOS  LEVEL=1  AREA=1  SCALE=1  LENGTH=1e-4 mm  WIDTH=1e-4 mm  AD=0 m^2  AS=0 m^2  PD=0 m  PS=0 m  NRD=1  NRS=1  RD=0.01 Ohm  RS=1e-4 Ohm  RSH=NaN Ohm  VTO=0 V  KP=2e-5 A/V^2  GAMMA=0 V^0.50000  PHI=0.6 V  LAMBDA=0 1/V  IS=1e-14 A  N=1  JS=0 A/m^2  DELTA=0  VMAX=0 m/s  NFS=0 1/cm^2  ETA=0  THETA=0 1/V  KAPPA=0.2  Ci_param=ee.enum.intrinsicCapacitance.none  Cov_param=1  CGSO=0 F/m  CGDO=0 F/m  CGBO=0 F/m  C_param=1  CBD=0 F  CBS=0 F  PB=0.8 V  CJ=0 F/m^2  MJ=0.5  CJSW=0 F/m  MJSW=0.5  FC=0.5  IC_given=1  ICVDS=0 V  ICVGS=0 V  ICVBS=0 V  TOX=1e-7 m  LD=0 m  U0=600 cm^2/s/V  NSUB=NaN 1/cm^3  TPG=1  NSS=0 1/cm^2  XJ=0 m  T_param=1  TFIXED=300.15 K  TMEAS=300.15 K  TOFFSET=0 K  UEXP=0  UCRIT=1e+4 V/cm  NEFF=1  MTYPE=1
      settings: InternalSimscapePortConfiguration="{\"Bottom\":[],\"Left\":[{\"id\":\"gx\",\"label\":\"\",\"type\":\"foundation.electrical.electrical\"}],\"Right\":[{\"id\":\"dx\",\"label\":\"\",\"type\":\"foundation.electrical.electrical\"},{\"id\":\"bx\",\"label\":\"\",\"type\":\"foundation.electrical.electrical\"},{\"id\":\"sx\",\"label\":\"\",\"type\":\"foundation.electrical.electrical\"}],\"Top\":[]}"
  SPICE PMOS8 : ee_lib/Additional Components/SPICE Semiconductors/SPICE PMOS  LEVEL=1  AREA=1  SCALE=1  LENGTH=1e-4 mm  WIDTH=1e-4 mm  AD=0 m^2  AS=0 m^2  PD=0 m  PS=0 m  NRD=1  NRS=1  RD=0.01 Ohm  RS=1e-4 Ohm  RSH=NaN Ohm  VTO=0 V  KP=2e-5 A/V^2  GAMMA=0 V^0.50000  PHI=0.6 V  LAMBDA=0 1/V  IS=1e-14 A  N=1  JS=0 A/m^2  DELTA=0  VMAX=0 m/s  NFS=0 1/cm^2  ETA=0  THETA=0 1/V  KAPPA=0.2  Ci_param=ee.enum.intrinsicCapacitance.none  Cov_param=1  CGSO=0 F/m  CGDO=0 F/m  CGBO=0 F/m  C_param=1  CBD=0 F  CBS=0 F  PB=0.8 V  CJ=0 F/m^2  MJ=0.5  CJSW=0 F/m  MJSW=0.5  FC=0.5  IC_given=1  ICVDS=0 V  ICVGS=0 V  ICVBS=0 V  TOX=1e-7 m  LD=0 m  U0=600 cm^2/s/V  NSUB=NaN 1/cm^3  TPG=1  NSS=0 1/cm^2  XJ=0 m  T_param=1  TFIXED=300.15 K  TMEAS=300.15 K  TOFFSET=0 K  UEXP=0  UCRIT=1e+4 V/cm  NEFF=1  MTYPE=-1
      settings: InternalSimscapePortConfiguration="{\"Bottom\":[],\"Left\":[{\"id\":\"gx\",\"label\":\"\",\"type\":\"foundation.electrical.electrical\"}],\"Right\":[{\"id\":\"dx\",\"label\":\"\",\"type\":\"foundation.electrical.electrical\"},{\"id\":\"bx\",\"label\":\"\",\"type\":\"foundation.electrical.electrical\"},{\"id\":\"sx\",\"label\":\"\",\"type\":\"foundation.electrical.electrical\"}],\"Top\":[]}"
  Conn1 : PMIOPort  Side=Right
  Conn2 : PMIOPort  Port=2  Side=Left
  connections:
  DC Voltage Source10/RConn1 -- Electrical Reference19/LConn1
  SPICE NMOS11/RConn1 -- Conn2/RConn1 -- SPICE PMOS8/RConn3
  Electrical Reference18/LConn1 -- DC Voltage Source11/RConn1
  DC Voltage Source11/LConn1 -- SPICE NMOS11/RConn2 -- SPICE NMOS11/RConn3
  DC Voltage Source10/LConn1 -- SPICE PMOS8/RConn1 -- SPICE PMOS8/RConn2
  Conn1/RConn1 -- SPICE NMOS11/LConn1 -- SPICE PMOS8/LConn1

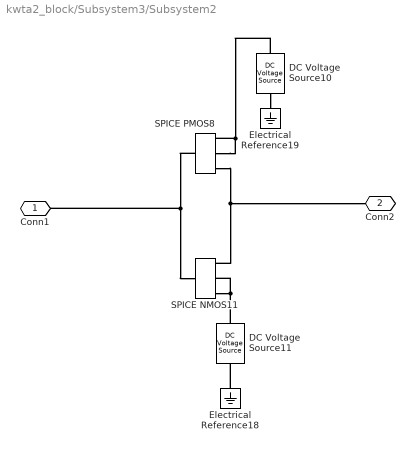
== system kwta2_block/Subsystem3/Subsystem2 ==
  DC Voltage Source10 : fl_lib/Electrical/Electrical Sources/DC Voltage Source  v0=5 V
  DC Voltage Source11 : fl_lib/Electrical/Electrical Sources/DC Voltage Source  v0=0 V
  Electrical Reference18 : fl_lib/Electrical/Electrical Elements/Electrical Reference
  Electrical Reference19 : fl_lib/Electrical/Electrical Elements/Electrical Reference
  SPICE NMOS11 : ee_lib/Additional Components/SPICE Semiconductors/SPICE NMOS  LEVEL=1  AREA=1  SCALE=1  LENGTH=1e-4 mm  WIDTH=1e-4 mm  AD=0 m^2  AS=0 m^2  PD=0 m  PS=0 m  NRD=1  NRS=1  RD=0.01 Ohm  RS=1e-4 Ohm  RSH=NaN Ohm  VTO=0 V  KP=2e-5 A/V^2  GAMMA=0 V^0.50000  PHI=0.6 V  LAMBDA=0 1/V  IS=1e-14 A  N=1  JS=0 A/m^2  DELTA=0  VMAX=0 m/s  NFS=0 1/cm^2  ETA=0  THETA=0 1/V  KAPPA=0.2  Ci_param=ee.enum.intrinsicCapacitance.none  Cov_param=1  CGSO=0 F/m  CGDO=0 F/m  CGBO=0 F/m  C_param=1  CBD=0 F  CBS=0 F  PB=0.8 V  CJ=0 F/m^2  MJ=0.5  CJSW=0 F/m  MJSW=0.5  FC=0.5  IC_given=1  ICVDS=0 V  ICVGS=0 V  ICVBS=0 V  TOX=1e-7 m  LD=0 m  U0=600 cm^2/s/V  NSUB=NaN 1/cm^3  TPG=1  NSS=0 1/cm^2  XJ=0 m  T_param=1  TFIXED=300.15 K  TMEAS=300.15 K  TOFFSET=0 K  UEXP=0  UCRIT=1e+4 V/cm  NEFF=1  MTYPE=1
      settings: InternalSimscapePortConfiguration="{\"Bottom\":[],\"Left\":[{\"id\":\"gx\",\"label\":\"\",\"type\":\"foundation.electrical.electrical\"}],\"Right\":[{\"id\":\"dx\",\"label\":\"\",\"type\":\"foundation.electrical.electrical\"},{\"id\":\"bx\",\"label\":\"\",\"type\":\"foundation.electrical.electrical\"},{\"id\":\"sx\",\"label\":\"\",\"type\":\"foundation.electrical.electrical\"}],\"Top\":[]}"
  SPICE PMOS8 : ee_lib/Additional Components/SPICE Semiconductors/SPICE PMOS  LEVEL=1  AREA=1  SCALE=1  LENGTH=1e-4 mm  WIDTH=1e-4 mm  AD=0 m^2  AS=0 m^2  PD=0 m  PS=0 m  NRD=1  NRS=1  RD=0.01 Ohm  RS=1e-4 Ohm  RSH=NaN Ohm  VTO=0 V  KP=2e-5 A/V^2  GAMMA=0 V^0.50000  PHI=0.6 V  LAMBDA=0 1/V  IS=1e-14 A  N=1  JS=0 A/m^2  DELTA=0  VMAX=0 m/s  NFS=0 1/cm^2  ETA=0  THETA=0 1/V  KAPPA=0.2  Ci_param=ee.enum.intrinsicCapacitance.none  Cov_param=1  CGSO=0 F/m  CGDO=0 F/m  CGBO=0 F/m  C_param=1  CBD=0 F  CBS=0 F  PB=0.8 V  CJ=0 F/m^2  MJ=0.5  CJSW=0 F/m  MJSW=0.5  FC=0.5  IC_given=1  ICVDS=0 V  ICVGS=0 V  ICVBS=0 V  TOX=1e-7 m  LD=0 m  U0=600 cm^2/s/V  NSUB=NaN 1/cm^3  TPG=1  NSS=0 1/cm^2  XJ=0 m  T_param=1  TFIXED=300.15 K  TMEAS=300.15 K  TOFFSET=0 K  UEXP=0  UCRIT=1e+4 V/cm  NEFF=1  MTYPE=-1
      settings: InternalSimscapePortConfiguration="{\"Bottom\":[],\"Left\":[{\"id\":\"gx\",\"label\":\"\",\"type\":\"foundation.electrical.electrical\"}],\"Right\":[{\"id\":\"dx\",\"label\":\"\",\"type\":\"foundation.electrical.electrical\"},{\"id\":\"bx\",\"label\":\"\",\"type\":\"foundation.electrical.electrical\"},{\"id\":\"sx\",\"label\":\"\",\"type\":\"foundation.electrical.electrical\"}],\"Top\":[]}"
  Conn1 : PMIOPort  Side=Right
  Conn2 : PMIOPort  Port=2  Side=Left
  connections:
  DC Voltage Source10/RConn1 -- Electrical Reference19/LConn1
  SPICE NMOS11/RConn1 -- Conn2/RConn1 -- SPICE PMOS8/RConn3
  Electrical Reference18/LConn1 -- DC Voltage Source11/RConn1
  DC Voltage Source11/LConn1 -- SPICE NMOS11/RConn2 -- SPICE NMOS11/RConn3
  DC Voltage Source10/LConn1 -- SPICE PMOS8/RConn1 -- SPICE PMOS8/RConn2
  Conn1/RConn1 -- SPICE NMOS11/LConn1 -- SPICE PMOS8/LConn1

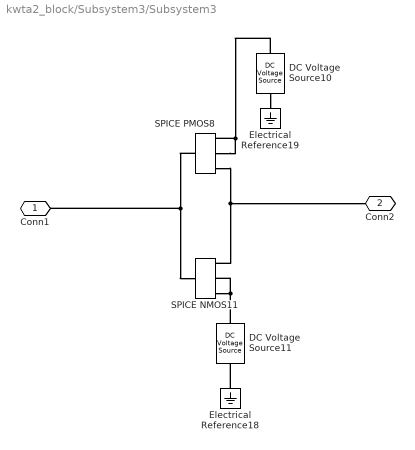
== system kwta2_block/Subsystem3/Subsystem3 ==
  DC Voltage Source10 : fl_lib/Electrical/Electrical Sources/DC Voltage Source  v0=5 V
  DC Voltage Source11 : fl_lib/Electrical/Electrical Sources/DC Voltage Source  v0=0 V
  Electrical Reference18 : fl_lib/Electrical/Electrical Elements/Electrical Reference
  Electrical Reference19 : fl_lib/Electrical/Electrical Elements/Electrical Reference
  SPICE NMOS11 : ee_lib/Additional Components/SPICE Semiconductors/SPICE NMOS  LEVEL=1  AREA=1  SCALE=1  LENGTH=1e-4 mm  WIDTH=1e-4 mm  AD=0 m^2  AS=0 m^2  PD=0 m  PS=0 m  NRD=1  NRS=1  RD=0.01 Ohm  RS=1e-4 Ohm  RSH=NaN Ohm  VTO=0 V  KP=2e-5 A/V^2  GAMMA=0 V^0.50000  PHI=0.6 V  LAMBDA=0 1/V  IS=1e-14 A  N=1  JS=0 A/m^2  DELTA=0  VMAX=0 m/s  NFS=0 1/cm^2  ETA=0  THETA=0 1/V  KAPPA=0.2  Ci_param=ee.enum.intrinsicCapacitance.none  Cov_param=1  CGSO=0 F/m  CGDO=0 F/m  CGBO=0 F/m  C_param=1  CBD=0 F  CBS=0 F  PB=0.8 V  CJ=0 F/m^2  MJ=0.5  CJSW=0 F/m  MJSW=0.5  FC=0.5  IC_given=1  ICVDS=0 V  ICVGS=0 V  ICVBS=0 V  TOX=1e-7 m  LD=0 m  U0=600 cm^2/s/V  NSUB=NaN 1/cm^3  TPG=1  NSS=0 1/cm^2  XJ=0 m  T_param=1  TFIXED=300.15 K  TMEAS=300.15 K  TOFFSET=0 K  UEXP=0  UCRIT=1e+4 V/cm  NEFF=1  MTYPE=1
      settings: InternalSimscapePortConfiguration="{\"Bottom\":[],\"Left\":[{\"id\":\"gx\",\"label\":\"\",\"type\":\"foundation.electrical.electrical\"}],\"Right\":[{\"id\":\"dx\",\"label\":\"\",\"type\":\"foundation.electrical.electrical\"},{\"id\":\"bx\",\"label\":\"\",\"type\":\"foundation.electrical.electrical\"},{\"id\":\"sx\",\"label\":\"\",\"type\":\"foundation.electrical.electrical\"}],\"Top\":[]}"
  SPICE PMOS8 : ee_lib/Additional Components/SPICE Semiconductors/SPICE PMOS  LEVEL=1  AREA=1  SCALE=1  LENGTH=1e-4 mm  WIDTH=1e-4 mm  AD=0 m^2  AS=0 m^2  PD=0 m  PS=0 m  NRD=1  NRS=1  RD=0.01 Ohm  RS=1e-4 Ohm  RSH=NaN Ohm  VTO=0 V  KP=2e-5 A/V^2  GAMMA=0 V^0.50000  PHI=0.6 V  LAMBDA=0 1/V  IS=1e-14 A  N=1  JS=0 A/m^2  DELTA=0  VMAX=0 m/s  NFS=0 1/cm^2  ETA=0  THETA=0 1/V  KAPPA=0.2  Ci_param=ee.enum.intrinsicCapacitance.none  Cov_param=1  CGSO=0 F/m  CGDO=0 F/m  CGBO=0 F/m  C_param=1  CBD=0 F  CBS=0 F  PB=0.8 V  CJ=0 F/m^2  MJ=0.5  CJSW=0 F/m  MJSW=0.5  FC=0.5  IC_given=1  ICVDS=0 V  ICVGS=0 V  ICVBS=0 V  TOX=1e-7 m  LD=0 m  U0=600 cm^2/s/V  NSUB=NaN 1/cm^3  TPG=1  NSS=0 1/cm^2  XJ=0 m  T_param=1  TFIXED=300.15 K  TMEAS=300.15 K  TOFFSET=0 K  UEXP=0  UCRIT=1e+4 V/cm  NEFF=1  MTYPE=-1
      settings: InternalSimscapePortConfiguration="{\"Bottom\":[],\"Left\":[{\"id\":\"gx\",\"label\":\"\",\"type\":\"foundation.electrical.electrical\"}],\"Right\":[{\"id\":\"dx\",\"label\":\"\",\"type\":\"foundation.electrical.electrical\"},{\"id\":\"bx\",\"label\":\"\",\"type\":\"foundation.electrical.electrical\"},{\"id\":\"sx\",\"label\":\"\",\"type\":\"foundation.electrical.electrical\"}],\"Top\":[]}"
  Conn1 : PMIOPort  Side=Right
  Conn2 : PMIOPort  Port=2  Side=Left
  connections:
  SPICE PMOS8/LConn1 -- SPICE NMOS11/LConn1 -- Conn1/RConn1
  SPICE PMOS8/RConn2 -- SPICE PMOS8/RConn1 -- DC Voltage Source10/LConn1
  SPICE NMOS11/RConn3 -- SPICE NMOS11/RConn2 -- DC Voltage Source11/LConn1
  Electrical Reference18/LConn1 -- DC Voltage Source11/RConn1
  SPICE PMOS8/RConn3 -- Conn2/RConn1 -- SPICE NMOS11/RConn1
  DC Voltage Source10/RConn1 -- Electrical Reference19/LConn1
